simulink model "Lab7"  (R2023a)
settings: Solver=VariableStepAuto  StartTime=0.0  StopTime=5  RelTol=1e-3
libraries: slpidlib x1
settings Model: Creator=lamiaa.zain  LastModifiedBy=lamiaa.zain

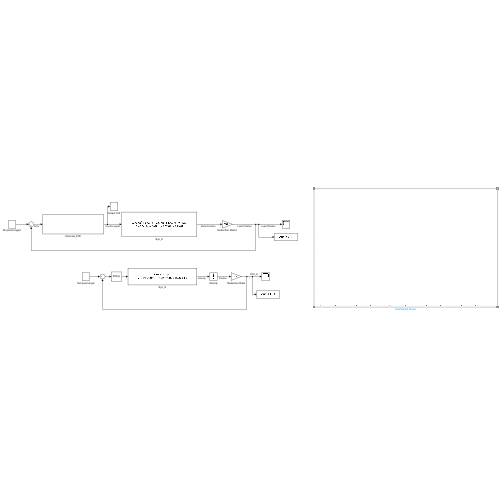
[thumbnail: Simulink's stored preview of the top-level diagram]
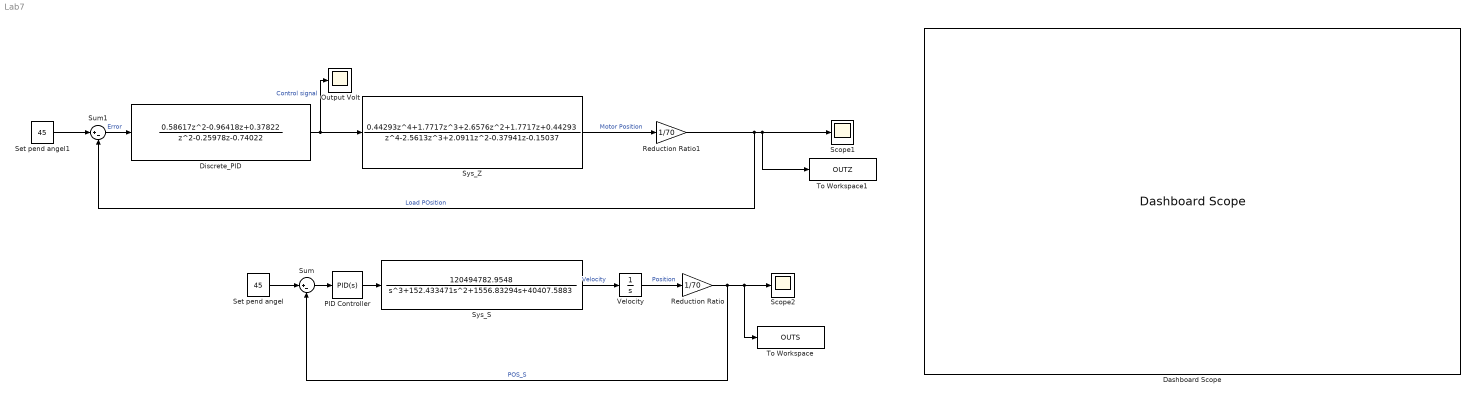
== system Lab7 ==
  Dashboard Scope : DashboardScope  Ymin=0  Ymax=0.2
  Discrete_PID : DiscreteTransferFcn  Numerator="[0.58617    -0.96418     0.37822]"  Denominator="[1    -0.25978    -0.74022]"  SampleTime=0.02
  Output Volt : Scope
  PID Controller : slpidlib/PID Controller  Controller=PID  Form=Parallel  TimeDomain=Continuous-time  UseExternalTs=off  SampleTime=0.01  IntegratorMethod=Forward Euler  FilterMethod=Forward Euler  ControllerParametersSource=internal  P=0.119488461149983  I=0.00611455847552309  UseKiTs=off  D=0.00536279599215705  N=669.887441993906  UseFilter=on  TunerSelectOption=Transfer Function Based (PID Tuner App)  InitialConditionSource=internal  InitialConditionForIntegrator=0  InitialConditionForFilter=0  DifferentiatorICPrevScaledInput=0  ExternalReset=none  TrackingMode=off  Kt=1  LimitOutput=off  SatLimitsSource=internal  UpperSaturationLimit=inf  LowerSaturationLimit=-inf  LinearizeAsGain=on  AntiWindupMode=none  Kb=1  LimitIntegrator=off  UpperIntegratorSaturationLimit=inf  LowerIntegratorSaturationLimit=-inf  POutMin=[]  POutMax=[]  IOutMin=[]  IOutMax=[]  DOutMin=[]  DOutMax=[]  NOutMin=[]  NOutMax=[]  SumOutMin=[]  SumOutMax=[]  SaturationOutMin=[]  SaturationOutMax=[]  PParamMin=[]  PParamMax=[]  IParamMin=[]  IParamMax=[]  DParamMin=[]  DParamMax=[]  NParamMin=[]  NParamMax=[]  KbParamMin=[]  KbParamMax=[]  KtParamMin=[]  KtParamMax=[]  KbOutMin=[]  KbOutMax=[]  KtOutMin=[]  KtOutMax=[]  IntegratorOutMin=[]  IntegratorOutMax=[]  FilterOutMin=[]  FilterOutMax=[]  SumI1OutMin=[]  SumI1OutMax=[]  SumI2OutMin=[]  SumI2OutMax=[]  SumI3OutMin=[]  SumI3OutMax=[]  SumI4OutMin=[]  SumI4OutMax=[]  SumDOutMin=[]  SumDOutMax=[]  DifferentiatorOutMin=[]  DifferentiatorOutMax=[]  FilterDiffOutCoefMin=[]  FilterDiffOutCoefMax=[]  ReciprocalOutMin=[]  ReciprocalOutMax=[]  SumDenOutMin=[]  SumDenOutMax=[]  SumNumOutMin=[]  SumNumOutMax=[]  DivideOutMin=[]  DivideOutMax=[]  UdiffTsProdOutMin=[]  UdiffTsProdOutMax=[]  NTsProdOutMin=[]  NTsProdOutMax=[]  UintegralTsProdOutMin=[]  UintegralTsProdOutMax=[]  UngainTsProdOutMin=[]  UngainTsProdOutMax=[]  ClampingZeroOutDataTypeStr=Inherit: Inherit via back propagation  ClampingZeroOutMin=[]  ClampingZeroOutMax=[]  FilterDenConstantOutDataTypeStr=Inherit: Inherit via back propagation  FilterDenConstantOutMin=[]  FilterDenConstantOutMax=[]  PCopyOutDataTypeStr=Inherit: Inherit via back propagation  PCopyOutMin=[]  PCopyOutMax=[]  NCopyOutDataTypeStr=Inherit: Inherit via back propagation  NCopyOutMin=[]  NCopyOutMax=[]  IntegratorContinuousStateAttributes=''  IntegratorStateMustResolveToSignalObject=off  IntegratorRTWStateStorageClass=Auto  FilterContinuousStateAttributes=''  FilterStateMustResolveToSignalObject=off  FilterRTWStateStorageClass=Auto  ParallelPVariant=InternalParameters  IdealPVariant=Disabled  IVariant=InternalParameters  DVariant=InternalParameters  IntegratorVariant=Continuous  SatVariant=Disabled  AWVariant=Passthrough  PCopyVariant=Disabled  TRVariant=Disabled  FdbkBlocksVariant=Forward  IdealPFdbkVariant=Disabled  SatFdbkVariant=Disabled  DerivativeFilterVariant=ContFilter  NVariant=InternalParameters  NCopyVariant=Disabled  FilterICVariant=InternalICsFilter  IntegratorICVariant=InternalICs  ExternalResetVariant=Disabled  TRSumVariant=Passthrough  SumFdbkVariant=Disabled  SumVariant=Sum_PID  TsampFilterVariant=InternalTs  TsampNgainVariant=Passthrough  TsampIntegralVariant=Disabled_SignalSpec  ExternalSaturationOutDataTypeStr=Inherit: Same as second input
  Reduction Ratio : Gain  Gain=1/70
  Reduction Ratio1 : Gain  Gain=1/70
  Scope1 : Scope
  Scope2 : Scope
  Set pend angel : Constant  Value=45
  Set pend angel1 : Constant  Value=45  SampleTime=0.02
  Sum : Sum  Inputs=|+-
  Sum1 : Sum  Inputs=|+-
  Sys_S : TransferFcn  Numerator="[0                   0                   0      120494782.9548]"  Denominator="[1      152.433471      1556.83294      40407.5883]"
  Sys_Z : DiscreteTransferFcn  Numerator="[0.44293      1.7717      2.6576      1.7717     0.44293]"  Denominator="[1     -2.5613      2.0911    -0.37941    -0.15037]"  SampleTime=0.02
  To Workspace : ToWorkspace  VariableName=OUTS  SaveFormat=Timeseries  SampleTime=-1
  To Workspace1 : ToWorkspace  VariableName=OUTZ  SaveFormat=Timeseries  SampleTime=-1
  Velocity : Integrator
  wires:
  Sum/1 -> PID Controller/1
  Set pend angel/1 -> Sum/1
  Sum1/1 -> Discrete_PID/1  "Error"
  Set pend angel1/1 -> Sum1/1
  Discrete_PID/1 -> Sys_Z/1, Output Volt/1  "Control signal"
  PID Controller/1 -> Sys_S/1
  Reduction Ratio1/1 -> Scope1/1, To Workspace1/1, Sum1/2  "Load POsition"
  Velocity/1 -> Reduction Ratio/1  "Position"
  Sys_Z/1 -> Reduction Ratio1/1  "Motor Position"
  Sys_S/1 -> Velocity/1  "Velocity"
  Reduction Ratio/1 -> Sum/2, To Workspace/1, Scope2/1  "POS_S"
